simulink model "eqestate"  (R2015a)
settings: Solver=ode45  StartTime=0.0  StopTime=50  RelTol=1e-3
values from neighbouring files (symbols this model uses):
  R = diag([Irw_par,Irw_par,Irw_par])    [ControlFeedback1.m]    (also in Equation_state.m)
undefined symbols (not defined in the file or in its folder): d, Equation_state
libraries: simulink x3
settings Model: Creator=Brayan  LastModifiedBy=Brayan

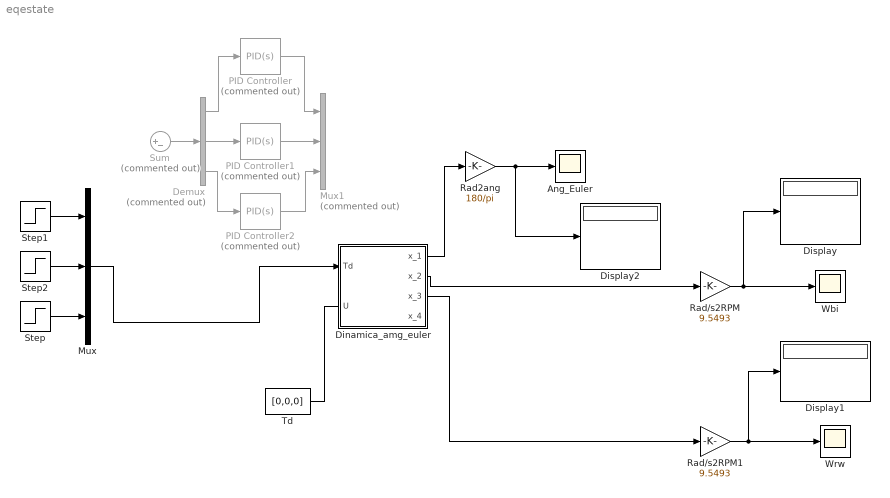
== system eqestate ==
  Ang_Euler : Scope
      settings: YMin=0  YMax=1
  Demux : Demux  Commented=on  Outputs=3
  Dinamica_amg_euler : Subsystem  mask{I=[10,10,10], InitialCondition=[0,0,0,0,0,0,0,0,0], Km=1, M=0.300, r=0.5}
      mask prompts: I "[Ix,Iy,Iz] :"; InitialCondition "Condiciones iniciales:"; M "Masa de ruedas de reaccion (M):"; r "Radio de ruedas de reaccion (r):"
      mask TypeOptions I: I/Value
      mask TypeOptions InitialCondition: Integrator1/InitialCondition
      mask TypeOptions Km: Km/Value
  Display : Display
  Display1 : Display
  Display2 : Display
  Mux : Mux  Inputs=3
  Mux1 : Mux  Commented=on  Inputs=3
  PID Controller : simulink/Continuous/PID Controller  Commented=on  Controller=PID  TimeDomain=Continuous-time  SampleTime=-1  IntegratorMethod=Forward Euler  FilterMethod=Forward Euler  Form=Parallel  UseFilter=on  ControllerParametersSource=internal  P=-0.0961828527170485  I=-0.0105995771108511  D=-0.214843633842694  N=26.348974238367  InitialConditionSource=internal  InitialConditionForIntegrator=0  InitialConditionForFilter=0  ExternalReset=none  LimitOutput=off  UpperSaturationLimit=inf  LowerSaturationLimit=-inf  LinearizeAsGain=on  AntiWindupMode=none  Kb=1  TrackingMode=off  Kt=1  PParamMin=[]  PParamMax=[]  IParamMin=[]  IParamMax=[]  DParamMin=[]  DParamMax=[]  NParamMin=[]  NParamMax=[]  KbParamMin=[]  KbParamMax=[]  KtParamMin=[]  KtParamMax=[]  POutMin=[]  POutMax=[]  IOutMin=[]  IOutMax=[]  DOutMin=[]  DOutMax=[]  NOutMin=[]  NOutMax=[]  KbOutMin=[]  KbOutMax=[]  KtOutMin=[]  KtOutMax=[]  IntegratorOutMin=[]  IntegratorOutMax=[]  FilterOutMin=[]  FilterOutMax=[]  SumOutMin=[]  SumOutMax=[]  SumI1OutMin=[]  SumI1OutMax=[]  SumI2OutMin=[]  SumI2OutMax=[]  SumI3OutMin=[]  SumI3OutMax=[]  SumDOutMin=[]  SumDOutMax=[]  SaturationOutMin=[]  SaturationOutMax=[]  IntegratorContinuousStateAttributes=''  IntegratorStateMustResolveToSignalObject=off  IntegratorRTWStateStorageClass=Auto  FilterContinuousStateAttributes=''  FilterStateMustResolveToSignalObject=off  FilterRTWStateStorageClass=Auto  DifferentiatorICPrevScaledInput=0  DifferentiatorOutMin=[]  DifferentiatorOutMax=[]
  PID Controller1 : simulink/Continuous/PID Controller  Commented=on  Controller=PID  TimeDomain=Continuous-time  SampleTime=-1  IntegratorMethod=Forward Euler  FilterMethod=Forward Euler  Form=Parallel  UseFilter=on  ControllerParametersSource=internal  P=-0.0961828527170485  I=-0.0105995771108511  D=-0.214843633842694  N=26.348974238367  InitialConditionSource=internal  InitialConditionForIntegrator=0  InitialConditionForFilter=0  ExternalReset=none  LimitOutput=off  UpperSaturationLimit=inf  LowerSaturationLimit=-inf  LinearizeAsGain=on  AntiWindupMode=none  Kb=1  TrackingMode=off  Kt=1  PParamMin=[]  PParamMax=[]  IParamMin=[]  IParamMax=[]  DParamMin=[]  DParamMax=[]  NParamMin=[]  NParamMax=[]  KbParamMin=[]  KbParamMax=[]  KtParamMin=[]  KtParamMax=[]  POutMin=[]  POutMax=[]  IOutMin=[]  IOutMax=[]  DOutMin=[]  DOutMax=[]  NOutMin=[]  NOutMax=[]  KbOutMin=[]  KbOutMax=[]  KtOutMin=[]  KtOutMax=[]  IntegratorOutMin=[]  IntegratorOutMax=[]  FilterOutMin=[]  FilterOutMax=[]  SumOutMin=[]  SumOutMax=[]  SumI1OutMin=[]  SumI1OutMax=[]  SumI2OutMin=[]  SumI2OutMax=[]  SumI3OutMin=[]  SumI3OutMax=[]  SumDOutMin=[]  SumDOutMax=[]  SaturationOutMin=[]  SaturationOutMax=[]  IntegratorContinuousStateAttributes=''  IntegratorStateMustResolveToSignalObject=off  IntegratorRTWStateStorageClass=Auto  FilterContinuousStateAttributes=''  FilterStateMustResolveToSignalObject=off  FilterRTWStateStorageClass=Auto  DifferentiatorICPrevScaledInput=0  DifferentiatorOutMin=[]  DifferentiatorOutMax=[]
  PID Controller2 : simulink/Continuous/PID Controller  Commented=on  Controller=PID  TimeDomain=Continuous-time  SampleTime=-1  IntegratorMethod=Forward Euler  FilterMethod=Forward Euler  Form=Parallel  UseFilter=on  ControllerParametersSource=internal  P=-0.0961828527170485  I=-0.0105995771108511  D=-0.214843633842694  N=26.348974238367  InitialConditionSource=internal  InitialConditionForIntegrator=0  InitialConditionForFilter=0  ExternalReset=none  LimitOutput=off  UpperSaturationLimit=inf  LowerSaturationLimit=-inf  LinearizeAsGain=on  AntiWindupMode=none  Kb=1  TrackingMode=off  Kt=1  PParamMin=[]  PParamMax=[]  IParamMin=[]  IParamMax=[]  DParamMin=[]  DParamMax=[]  NParamMin=[]  NParamMax=[]  KbParamMin=[]  KbParamMax=[]  KtParamMin=[]  KtParamMax=[]  POutMin=[]  POutMax=[]  IOutMin=[]  IOutMax=[]  DOutMin=[]  DOutMax=[]  NOutMin=[]  NOutMax=[]  KbOutMin=[]  KbOutMax=[]  KtOutMin=[]  KtOutMax=[]  IntegratorOutMin=[]  IntegratorOutMax=[]  FilterOutMin=[]  FilterOutMax=[]  SumOutMin=[]  SumOutMax=[]  SumI1OutMin=[]  SumI1OutMax=[]  SumI2OutMin=[]  SumI2OutMax=[]  SumI3OutMin=[]  SumI3OutMax=[]  SumDOutMin=[]  SumDOutMax=[]  SaturationOutMin=[]  SaturationOutMax=[]  IntegratorContinuousStateAttributes=''  IntegratorStateMustResolveToSignalObject=off  IntegratorRTWStateStorageClass=Auto  FilterContinuousStateAttributes=''  FilterStateMustResolveToSignalObject=off  FilterRTWStateStorageClass=Auto  DifferentiatorICPrevScaledInput=0  DifferentiatorOutMin=[]  DifferentiatorOutMax=[]
  Rad/s2RPM : Gain  Gain=9.5493
  Rad/s2RPM1 : Gain  Gain=9.5493
  Rad2ang : Gain  Gain=180/pi
  Step : Step  After=0  SampleTime=0
  Step1 : Step  Before=1  After=0  SampleTime=0
  Step2 : Step  After=0  SampleTime=0
  Sum : Sum  Commented=on  Inputs=|+-
  Td : Constant  Value=[0,0,0]
  Wbi : Scope
      settings: SaveName=ScopeData2
  "Wrw " : Scope
  wires:
  Step1/1 -> Mux/1
  Step2/1 -> Mux/2
  Step/1 -> Mux/3
  Td/1 -> ?
  Dinamica_amg_euler/1(x_1) -> Rad2ang/1
  Rad2ang/1 -> Display2/1, Ang_Euler/1
  Dinamica_amg_euler/2("x_2 ") -> Rad/s2RPM/1
  Dinamica_amg_euler/3(x_3) -> Rad/s2RPM1/1
  Rad/s2RPM/1 -> Display/1, Wbi/1
  Rad/s2RPM1/1 -> Display1/1, "Wrw "/1
  Sum/1 -> Demux/1
  Demux/1 -> PID Controller/1
  PID Controller/1 -> Mux1/1
  Demux/2 -> PID Controller1/1
  PID Controller1/1 -> Mux1/2
  Demux/3 -> PID Controller2/1
  PID Controller2/1 -> Mux1/3
  Mux/1 -> Dinamica_amg_euler/1(Td)

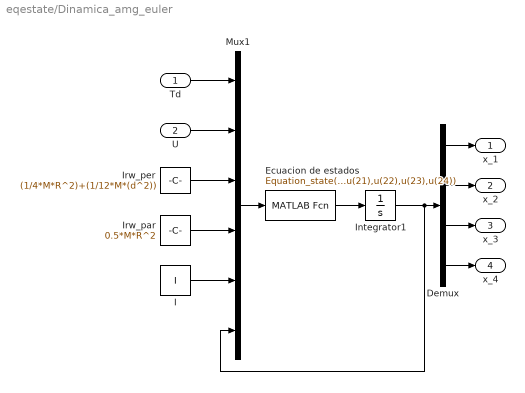
== system eqestate/Dinamica_amg_euler ==
  Td : Inport
  U : Inport  Port=2
  Demux : Demux
  Ecuacion de estados : MATLABFcn  MATLABFcn=Equation_state(u(1),u(2),u(3),u(4),u(5),u(6),u(7),u(8),u(9),u(10),u(11),u(12),u(13),u(14),u(15),u(16),u(17),u(18),u(19),u(20),u(21),u(22),u(23),u(24))
  I : Constant  Value=I
  Integrator1 : Integrator  InitialCondition=InitialCondition
  Irw_par : Constant  Value=0.5*M*R^2
  Irw_per : Constant  Value=(1/4*M*R^2)+(1/12*M*(d^2))
  Mux1 : Mux  Inputs=6
  x_1 : Outport
  "x_2 " : Outport  Port=2
  x_3 : Outport  Port=3
  x_4 : Outport  Port=4
  wires:
  Demux/1 -> x_1/1
  Integrator1/1 -> Mux1/6, Demux/1
  Demux/3 -> x_3/1
  Demux/2 -> "x_2 "/1
  Td/1 -> Mux1/1
  Ecuacion de estados/1 -> Integrator1/1
  Mux1/1 -> Ecuacion de estados/1
  U/1 -> Mux1/2
  Irw_par/1 -> Mux1/4
  Demux/4 -> x_4/1
  Irw_per/1 -> Mux1/3
  I/1 -> Mux1/5
